simulink model "test2"  (R2018b)
settings: Solver=FixedStepAuto  StartTime=0.0  StopTime=20  FixedStep=0.001  RelTol=1e-3
settings Model: Creator=User  LastModifiedBy=User

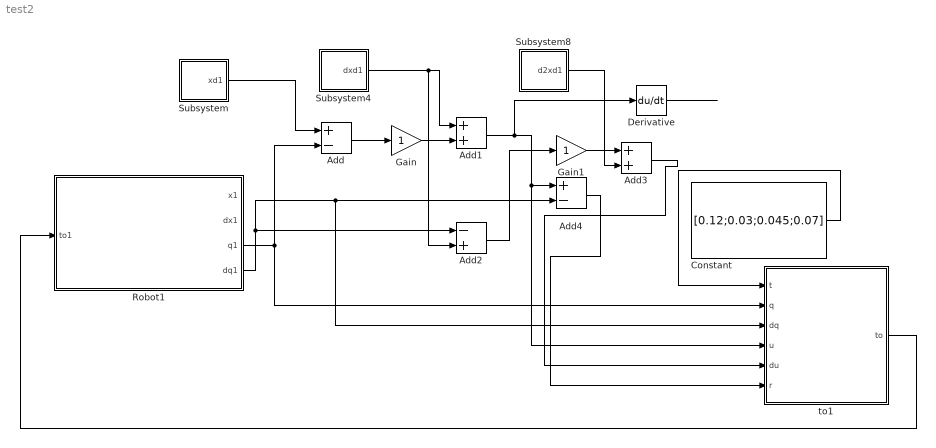
== system test2 ==
  Add : Sum  Inputs=+-
  Add1 : Sum
  Add2 : Sum  Inputs=-+
  Add3 : Sum
  Add4 : Sum  Inputs=+-
  Constant : Constant  Value=[0.12;0.03;0.045;0.07]
  Derivative : Derivative
  Gain : Gain
  Gain1 : Gain
  Robot1 : Subsystem
  Subsystem : Subsystem
  Subsystem4 : Subsystem
  Subsystem8 : Subsystem
  to1 : MATLAB Function  TreatAsAtomicUnit=on
  wires:
  to1/1(to) -> Robot1/1(to1)
  Add3/1 -> to1/5(du)
  Subsystem/1(xd1) -> Add/1
  Constant/1 -> to1/1(t)
  Gain1/1 -> Add3/1
  Add1/1 -> Derivative/1, Add4/1, to1/4(u)
  Add2/1 -> Gain1/1
  Robot1/4(dq1) -> to1/3(dq), Add4/2, Add2/1
  Add/1 -> Gain/1
  Subsystem4/1(dxd1) -> Add2/2, Add1/1
  Add4/1 -> to1/6(r)
  Robot1/3(q1) -> to1/2(q), Add/2
  Subsystem8/1(d2xd1) -> Add3/2
  Gain/1 -> Add1/2
  Derivative/1 -> ?

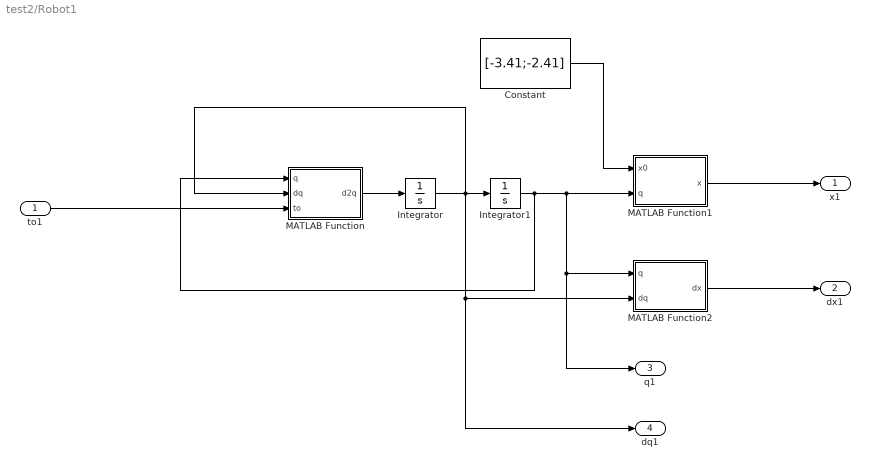
== system test2/Robot1 ==
  to1 : Inport
  Constant : Constant  Value=[-3.41;-2.41]
  Integrator : Integrator  InitialCondition=[0;0]
  Integrator1 : Integrator  InitialCondition=[pi/6;pi/6]
  MATLAB Function : MATLAB Function  TreatAsAtomicUnit=on
  MATLAB Function1 : MATLAB Function  TreatAsAtomicUnit=on
  MATLAB Function2 : MATLAB Function  TreatAsAtomicUnit=on
  x1 : Outport
  dx1 : Outport  Port=2
  q1 : Outport  Port=3
  dq1 : Outport  Port=4
  wires:
  to1/1 -> MATLAB Function/3(to)
  MATLAB Function/1(d2q) -> Integrator/1
  Integrator/1 -> dq1/1, MATLAB Function2/2(dq), MATLAB Function/2(dq), Integrator1/1
  Integrator1/1 -> q1/1, MATLAB Function2/1(q), MATLAB Function1/2(q), MATLAB Function/1(q)
  MATLAB Function1/1(x) -> x1/1
  Constant/1 -> MATLAB Function1/1(x0)
  MATLAB Function2/1(dx) -> dx1/1

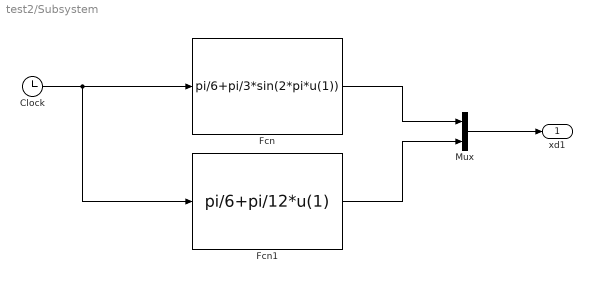
== system test2/Subsystem ==
  Clock : Clock
  Fcn : Fcn  Expr=pi/6+pi/3*sin(2*pi*u(1))
  Fcn1 : Fcn  Expr=pi/6+pi/12*u(1)
  Mux : Mux  Inputs=2
  xd1 : Outport
  wires:
  Clock/1 -> Fcn1/1, Fcn/1
  Fcn/1 -> Mux/1
  Fcn1/1 -> Mux/2
  Mux/1 -> xd1/1

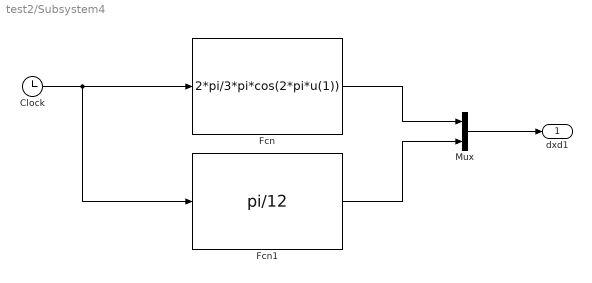
== system test2/Subsystem4 ==
  Clock : Clock
  Fcn : Fcn  Expr=2*pi/3*pi*cos(2*pi*u(1))
  Fcn1 : Fcn  Expr=pi/12
  Mux : Mux  Inputs=2
  dxd1 : Outport
  wires:
  Mux/1 -> dxd1/1
  Fcn1/1 -> Mux/2
  Fcn/1 -> Mux/1
  Clock/1 -> Fcn/1, Fcn1/1

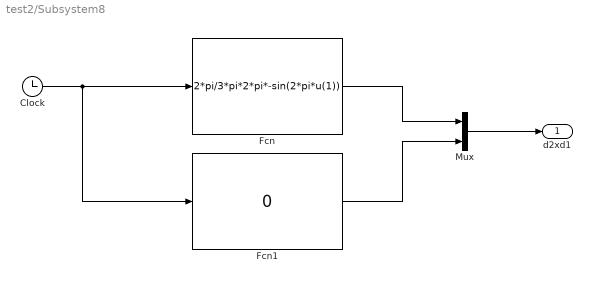
== system test2/Subsystem8 ==
  Clock : Clock
  Fcn : Fcn  Expr=2*pi/3*pi*2*pi*-sin(2*pi*u(1))
  Fcn1 : Fcn  Expr=0
  Mux : Mux  Inputs=2
  d2xd1 : Outport
  wires:
  Clock/1 -> Fcn1/1, Fcn/1
  Fcn/1 -> Mux/1
  Fcn1/1 -> Mux/2
  Mux/1 -> d2xd1/1

== matlab function test2/Robot1/MATLAB Function1 ==
  data: x0 input; x output; q input
function x = fcn(x0,q)
q1=q(1);
q2=q(2);
x=x0+[0.3*cos(q1)+0.3*cos(q1+q2);0.3*sin(q1)+0.3*sin(q1+q2)];
end

== matlab function test2/Robot1/MATLAB Function ==
  data: q input; d2q output; dq input; to input
function d2q = fcn(q,dq,to)
m1=1;
m2=1;
l1=0.3;
l2=0.3;
t1=1/3*m1*l1^2+m2*l1^2;
t2=1/3*m2*l2^2;
t3=1/2*m2*l1*l2;
t4=0.07;
q2=q(2);
M=[t1+t2+2*t3*cos(q2) t2+t3*cos(q2);
    t2+t3*cos(q2) t2];
dq1=dq(1);
dq2=dq(2);
V=[-dq2*dq1*t3*sin(q2)-(dq1+dq2)*dq2*t3*sin(q2)+t4*dq1;
    dq1^2*t3*sin(q2)+t4*dq2];
d2q=M\(to-V);
end

== matlab function test2/Robot1/MATLAB Function2 ==
  data: q input; dq input; dx output
function dx = fcn(q,dq)
q1=q(1);
q2=q(2);
J=[-0.3*sin(q1)-0.3*sin(q1+q2) -0.3*sin(q1+q2);
    0.3*cos(q1)+0.3*cos(q1+q2) 0.3*cos(q1+q2)];
dx=J*dq;
end

== matlab function test2/to1 ==
  data: t input; q input; dq input; u input; to output; du input; r input
function to = fcn(t,q,dq,u,du,r)
t1=t(1);
t2=t(2);
t3=t(3);
t4=t(4);
q2=q(2);
Hq=[t1+t2+2*t3*cos(q2) t2+t3*cos(q2);
    t2+t3*cos(q2) t2];
dq1=dq(1);
dq2=dq(2);
Cq=[-dq2*t3*sin(q2) -(dq1+dq2)*t3*sin(q2);
    dq1*t3*sin(q2) 0];
Fq=[t4*dq1;t4*dq2];
to=Hq*du+Cq*u+Fq+1*r;
end
